simulink model "ANN"  (R2021b)
settings: Solver=FixedStepDiscrete  StartTime=0.0  StopTime=1  RelTol=1e-3
undefined symbols (not defined in the file or in its folder): alpha, b1, b2, b3, input, target, train, w1, w2, w3
Description:
  | Symmetric FIR Filter
  | This example shows how to use HDL Coder(TM) to check, generate,
  | and verify HDL for a fixed-point symmetric FIR filter.
settings Model: DataTypeOverride=Off  Creator=The MathWorks, Inc.  LastModifiedBy=bogru
settings SolverCC: AlgebraicLoopSolver=TrustRegion
settings DataIOCC: LimitDataPoints=on  SaveFormat=Array  SaveOutput=off  SignalLogging=off  SaveTime=off  ReturnWorkspaceOutputs=off  SignalLoggingName=logsOut
settings OptimizationCC: BlockReduction=off  BooleanDataType=off  ConditionallyExecuteInputs=off  DefaultParameterBehavior=Inlined  InheritOutputTypeSmallerThanSingle=on  InlineInvariantSignals=on  ExpressionDepthLimit=2147483647  InitFltsAndDblsToZero=on  LifeSpan=inf  BufferReusableBoundary=off
settings DebuggingCC: AlgebraicLoopMsg=error  SaveWithParameterizedLinksMsg=none  UnderspecifiedInitializationDetection=Classic  MergeDetectMultiDrivingBlocksExec=none  CheckExecutionContextPreStartOutputMsg=on  SignalResolutionControl=TryResolveAllWithWarning  MultiTaskDSMMsg=warning  MultiTaskCondExecSysMsg=none  SingleTaskRateTransMsg=error  IntegerOverflowMsg=none  ParameterPrecisionLossMsg=none  FcnCallInpInsideContextMsg=warning  BusObjectLabelMismatch=none  StateNameClashWarn=warning  SFUnexpectedBacktrackingDiag=warning  SFNoUnconditionalDefaultTransitionDiag=warning  SFExecutionAtInitializationDiag=none  SFMachineParentedDataDiag=warning  IntegerSaturationMsg=none  ArithmeticOperatorsInVariantConditions=warning
settings HardwareCC: ProdBitPerPointer=32  ProdBitPerSizeT=32  ProdBitPerPtrDiffT=32  ProdLargestAtomicFloat=None  ProdIntDivRoundTo=Undefined  ProdEndianess=Unspecified  ProdWordSize=32  ProdHWDeviceType=ASIC/FPGA  TargetUnknown=on  ProdEqTarget=off
settings ModelReferenceCC: PropagateSignalLabelsOutOfModel=off
settings SFSimCC: SimUseLocalCustomCode=off  CustomCodeUndefinedFunction=UseInterfaceOnly
settings RTWCC: RTWUseLocalCustomCode=off
settings CodeAppCC: StateflowObjectComments=on
settings GRTTargetCC: TargetFcnLib=ansi_tfl_tmw.mat  TargetLangStandard=C89/C90 (ANSI)  CombineOutputUpdateFcns=off  GRTInterface=on
settings ConfigComp: CovMetricSettings=dw  CovSaveCumulativeToWorkspaceVar=on  CovSaveSingleToWorkspaceVar=on  CovExternalEMLEnable=off

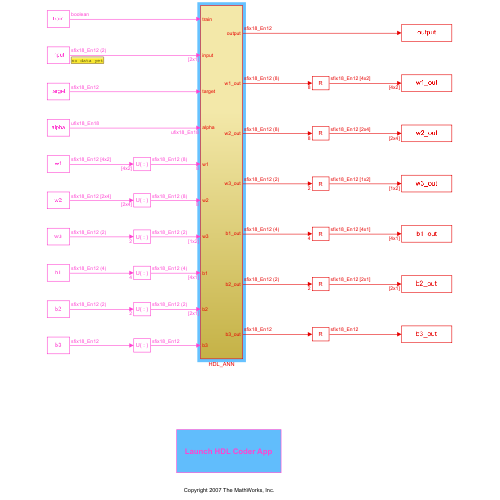
[thumbnail: Simulink's stored preview of the top-level diagram]
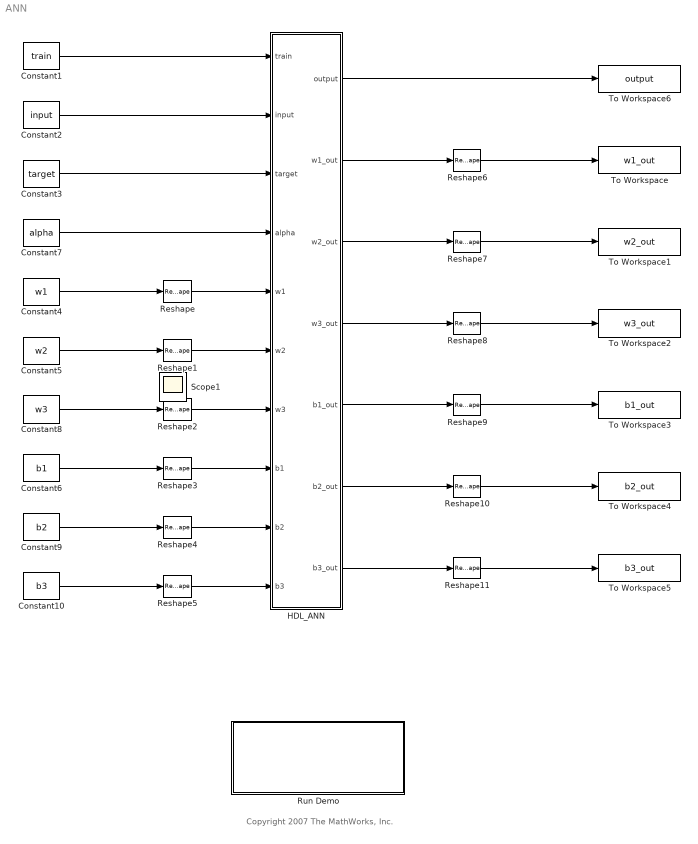
== system ANN ==
  note: Copyright 2007 The MathWorks, Inc.
  Constant1 : Constant  Value=train  OutDataTypeStr=boolean
  Constant10 : Constant  Value=b3  OutDataTypeStr=fixdt(1,18,12)
  Constant2 : Constant  Value=input  OutDataTypeStr=fixdt(1,18,12)
  Constant3 : Constant  Value=target  OutDataTypeStr=fixdt(1,18,12)
  Constant4 : Constant  Value=w1  OutDataTypeStr=fixdt(1,18,12)
  Constant5 : Constant  Value=w2  OutDataTypeStr=fixdt(1,18,12)
  Constant6 : Constant  Value=b1  OutDataTypeStr=fixdt(1,18,12)
  Constant7 : Constant  Value=alpha  OutDataTypeStr=fixdt(0,18,18)
  Constant8 : Constant  Value=w3  OutDataTypeStr=fixdt(1,18,12)
  Constant9 : Constant  Value=b2  OutDataTypeStr=fixdt(1,18,12)
  HDL_ANN : Subsystem
  Reshape{,1..5} (6 alike) : Reshape
  Reshape10 : Reshape  OutputDimensionality=Customize  OutputDimensions=[2 1]
  Reshape11 : Reshape  OutputDimensionality=Customize  OutputDimensions=[1 1]
  Reshape6 : Reshape  OutputDimensionality=Customize  OutputDimensions=[4 2]
  Reshape7 : Reshape  OutputDimensionality=Customize  OutputDimensions=[2 4]
  Reshape8 : Reshape  OutputDimensionality=Customize  OutputDimensions=[1 2]
  Reshape9 : Reshape  OutputDimensionality=Customize  OutputDimensions=[4 1]
  Run Demo : Subsystem
      settings: OpenFcn=hdltoolstrip(bdroot)
      mask Display: disp('Launch HDL Coder App')
  To Workspace : ToWorkspace  VariableName=w1_out  SampleTime=-1
      settings: MaxDataPoints=1
  To Workspace1 : ToWorkspace  VariableName=w2_out  SampleTime=-1
      settings: MaxDataPoints=1
  To Workspace2 : ToWorkspace  VariableName=w3_out  SampleTime=-1
      settings: MaxDataPoints=1
  To Workspace3 : ToWorkspace  VariableName=b1_out  SampleTime=-1
      settings: MaxDataPoints=1
  To Workspace4 : ToWorkspace  VariableName=b2_out  SampleTime=-1
      settings: MaxDataPoints=1
  To Workspace5 : ToWorkspace  VariableName=b3_out  SampleTime=-1
      settings: MaxDataPoints=1  Save2DSignal=2-D array (concatenate along first dimension)
  To Workspace6 : ToWorkspace  VariableName=output  SampleTime=-1
      settings: MaxDataPoints=1  Save2DSignal=2-D array (concatenate along first dimension)
  Scope1 : Scope
  wires:
  HDL_ANN/1(output) -> To Workspace6/1
  Constant7/1 -> HDL_ANN/4(alpha)
  Constant1/1 -> HDL_ANN/1(train)
  Constant3/1 -> HDL_ANN/3(target)
  Constant2/1 -> HDL_ANN/2(input)
  Constant4/1 -> Reshape/1
  Constant10/1 -> Reshape5/1
  Constant9/1 -> Reshape4/1
  Constant6/1 -> Reshape3/1
  Constant8/1 -> Reshape2/1
  Constant5/1 -> Reshape1/1
  HDL_ANN/2(w1_out) -> Reshape6/1
  Reshape/1 -> HDL_ANN/5(w1)
  Reshape1/1 -> HDL_ANN/6(w2)
  Reshape2/1 -> HDL_ANN/7(w3)
  Reshape3/1 -> HDL_ANN/8(b1)
  Reshape4/1 -> HDL_ANN/9(b2)
  Reshape5/1 -> HDL_ANN/10(b3)
  Reshape6/1 -> To Workspace/1
  HDL_ANN/3(w2_out) -> Reshape7/1
  Reshape7/1 -> To Workspace1/1
  HDL_ANN/4(w3_out) -> Reshape8/1
  Reshape8/1 -> To Workspace2/1
  HDL_ANN/5(b1_out) -> Reshape9/1
  Reshape9/1 -> To Workspace3/1
  HDL_ANN/6(b2_out) -> Reshape10/1
  Reshape10/1 -> To Workspace4/1
  HDL_ANN/7(b3_out) -> Reshape11/1
  Reshape11/1 -> To Workspace5/1

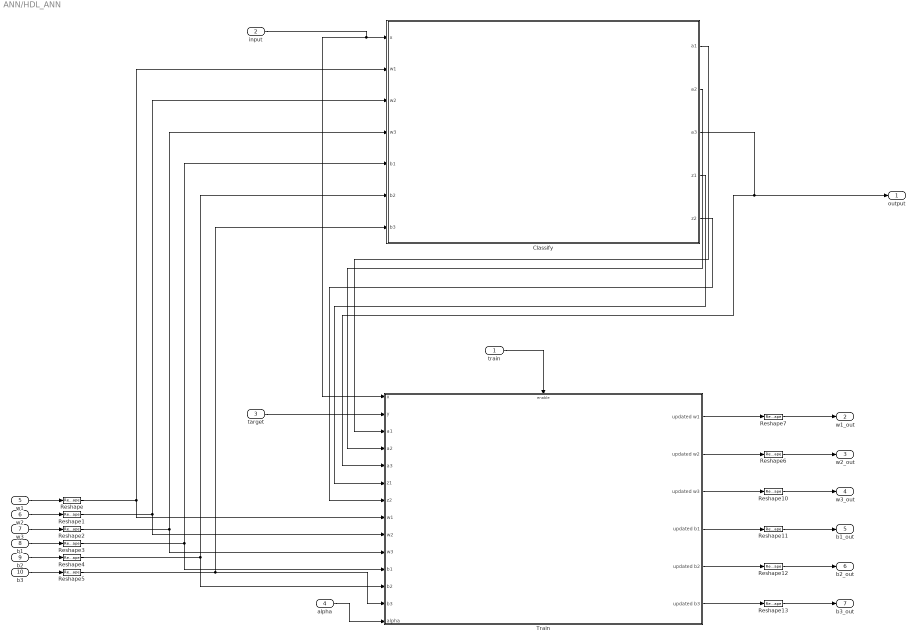
== system ANN/HDL_ANN ==
  train : Inport  SampleTime=1
  input : Inport  Port=2  PortDimensions=[2 1]  SampleTime=1
  target : Inport  Port=3  SampleTime=1
  alpha : Inport  Port=4  OutDataTypeStr=fixdt(0, 18, 18)  SampleTime=1
  w1 : Inport  Port=5  SampleTime=1
  w2 : Inport  Port=6  SampleTime=1
  w3 : Inport  Port=7  PortDimensions=[1 2]  SampleTime=1
  b1 : Inport  Port=8  PortDimensions=[4 1]  SampleTime=1
  b2 : Inport  Port=9  PortDimensions=[2 1]  SampleTime=1
  b3 : Inport  Port=10  PortDimensions=[1 1]  SampleTime=1
  Classify : Subsystem  TreatAsAtomicUnit=on
  Reshape : Reshape  OutputDimensionality=Customize  OutputDimensions=[4 2]
  Reshape1 : Reshape  OutputDimensionality=Customize  OutputDimensions=[2 4]
  Reshape{6..7,10..13} (6 alike) : Reshape  OutputDimensions=[4 2]
  Reshape2 : Reshape  OutputDimensionality=Customize  OutputDimensions=[1 2]
  Reshape3 : Reshape  OutputDimensionality=Customize  OutputDimensions=[4 1]
  Reshape4 : Reshape  OutputDimensionality=Customize  OutputDimensions=[2 1]
  Reshape5 : Reshape  OutputDimensionality=Customize  OutputDimensions=[1 1]
  Train : Subsystem  TreatAsAtomicUnit=on
  output : Outport
  w1_out : Outport  Port=2
  w2_out : Outport  Port=3
  w3_out : Outport  Port=4
  b1_out : Outport  Port=5
  b2_out : Outport  Port=6
  b3_out : Outport  Port=7
  wires:
  alpha/1 -> Train/14(alpha)
  Classify/2(a2) -> Train/4(a2)
  Classify/1(a1) -> Train/3(a1)
  Classify/3(a3) -> output/1, Train/5(a3)
  input/1 -> Train/1(x), Classify/1(x)
  target/1 -> Train/2(y)
  train/1 -> Train/Enable
  b3/1 -> Reshape5/1
  b2/1 -> Reshape4/1
  b1/1 -> Reshape3/1
  w3/1 -> Reshape2/1
  w1/1 -> Reshape/1
  Train/6(updated b3) -> Reshape13/1
  Train/5(updated b2) -> Reshape12/1
  Train/4(updated b1) -> Reshape11/1
  Train/3(updated w3) -> Reshape10/1
  Train/2(updated w2) -> Reshape6/1
  Train/1(updated w1) -> Reshape7/1
  Reshape/1 -> Classify/2(w1), Train/8(w1)
  Reshape1/1 -> Classify/3(w2), Train/9(w2)
  Reshape2/1 -> Classify/4(w3), Train/10(w3)
  Reshape3/1 -> Classify/5(b1), Train/11(b1)
  Reshape4/1 -> Classify/6(b2), Train/12(b2)
  Reshape5/1 -> Classify/7(b3), Train/13(b3)
  Reshape7/1 -> w1_out/1
  Reshape6/1 -> w2_out/1
  Reshape10/1 -> w3_out/1
  Reshape11/1 -> b1_out/1
  Reshape12/1 -> b2_out/1
  Reshape13/1 -> b3_out/1
  w2/1 -> Reshape1/1
  Classify/4(z1) -> Train/6(z1)
  Classify/5(z2) -> Train/7(z2)

== system ANN/Run Demo ==

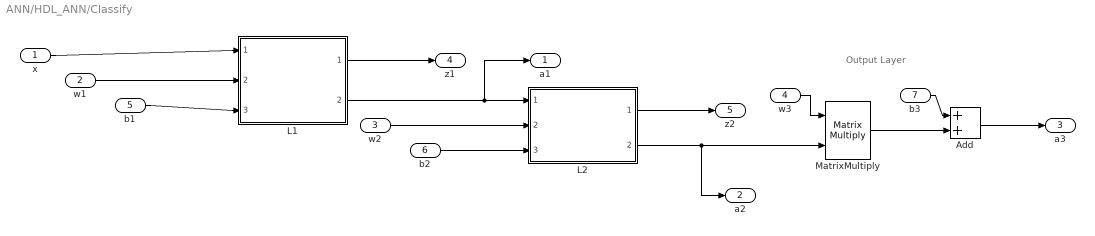
== system ANN/HDL_ANN/Classify ==
  note: Output Layer
  x : Inport
  w1 : Inport  Port=2
  w2 : Inport  Port=3
  w3 : Inport  Port=4
  b1 : Inport  Port=5
  b2 : Inport  Port=6
  b3 : Inport  Port=7
  Add : Sum  AccumDataTypeStr=fixdt(1,18,12)
  L1 : Subsystem  VariantControl=Choice  ReferencedSubsystem=ReLU_layer
  L2 : Subsystem  ReferencedSubsystem=ReLU_layer
  MatrixMultiply : Product  Multiplication=Matrix(*)  OutDataTypeStr=fixdt(1,18,12)
  a1 : Outport  InitialOutput=[0;0;0;0]
  a2 : Outport  Port=2  InitialOutput=[0;0]
  a3 : Outport  Port=3  InitialOutput=0
  z1 : Outport  Port=4  InitialOutput=[0;0;0;0]
  z2 : Outport  Port=5  InitialOutput=[0;0;0;0]
  wires:
  w2/1 -> L2/2
  b2/1 -> L2/3
  x/1 -> L1/1
  w1/1 -> L1/2
  b1/1 -> L1/3
  L1/1 -> z1/1
  L1/2 -> a1/1, L2/1
  L2/1 -> z2/1
  w3/1 -> MatrixMultiply/1
  L2/2 -> MatrixMultiply/2, a2/1
  b3/1 -> Add/1
  MatrixMultiply/1 -> Add/2
  Add/1 -> a3/1

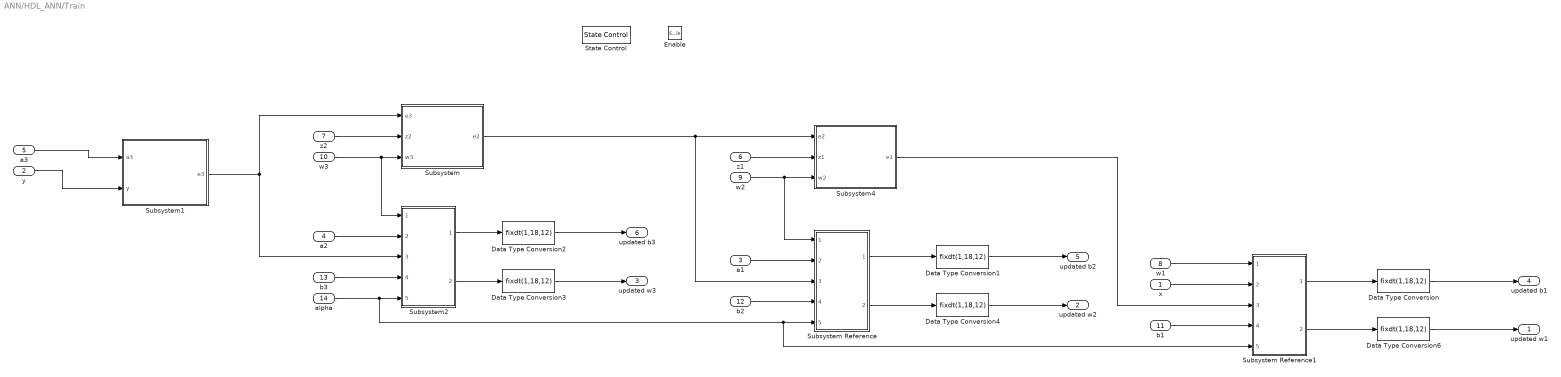
== system ANN/HDL_ANN/Train ==
  x : Inport
  y : Inport  Port=2
  a1 : Inport  Port=3
  a2 : Inport  Port=4
  a3 : Inport  Port=5
  z1 : Inport  Port=6
  z2 : Inport  Port=7
  w1 : Inport  Port=8
  w2 : Inport  Port=9
  w3 : Inport  Port=10
  b1 : Inport  Port=11
  b2 : Inport  Port=12
  b3 : Inport  Port=13
  alpha : Inport  Port=14
  Enable : EnablePort
  Data Type Conversion{,1..4,6} (6 alike) : DataTypeConversion  OutDataTypeStr=fixdt(1,18,12)
  State Control : StateControl  StateControl=Synchronous
  Subsystem : Subsystem
  Subsystem Reference : Subsystem  ReferencedSubsystem=WB_update
  Subsystem Reference1 : Subsystem  ReferencedSubsystem=WB_update
  Subsystem1 : Subsystem
  Subsystem2 : Subsystem  ReferencedSubsystem=WB_update
  Subsystem4 : Subsystem
  updated w1 : Outport  InitialOutput=[0 0; 0 0; 0 0; 0 0]
  updated w2 : Outport  Port=2  InitialOutput=[0 0 0 0; 0 0 0 0]
  updated w3 : Outport  Port=3  InitialOutput=[0 0]
  updated b1 : Outport  Port=4  InitialOutput=[0;0;0;0]
  updated b2 : Outport  Port=5  InitialOutput=[0;0]
  updated b3 : Outport  Port=6  InitialOutput=0
  wires:
  Data Type Conversion6/1 -> updated w1/1
  Subsystem4/1(e1) -> Subsystem Reference1/3
  Subsystem Reference1/2 -> Data Type Conversion6/1
  Data Type Conversion4/1 -> updated w2/1
  Subsystem/1(e2) -> Subsystem Reference/3, Subsystem4/1(e2)
  Data Type Conversion3/1 -> updated w3/1
  Subsystem2/2 -> Data Type Conversion3/1
  Data Type Conversion1/1 -> updated b2/1
  Data Type Conversion2/1 -> updated b3/1
  w2/1 -> Subsystem Reference/1, Subsystem4/3(w2)
  a1/1 -> Subsystem Reference/2
  b1/1 -> Subsystem Reference1/4
  b3/1 -> Subsystem2/4
  w1/1 -> Subsystem Reference1/1
  b2/1 -> Subsystem Reference/4
  Data Type Conversion/1 -> updated b1/1
  Subsystem Reference1/1 -> Data Type Conversion/1
  a2/1 -> Subsystem2/2
  x/1 -> Subsystem Reference1/2
  w3/1 -> Subsystem2/1, Subsystem/3(w3)
  Subsystem Reference/1 -> Data Type Conversion1/1
  Subsystem2/1 -> Data Type Conversion2/1
  alpha/1 -> Subsystem2/5, Subsystem Reference1/5, Subsystem Reference/5
  Subsystem Reference/2 -> Data Type Conversion4/1
  z1/1 -> Subsystem4/2(z1)
  z2/1 -> Subsystem/2(z2)
  Subsystem1/1(e3) -> Subsystem/1(e3), Subsystem2/3
  a3/1 -> Subsystem1/1(a3)
  y/1 -> Subsystem1/2(y)

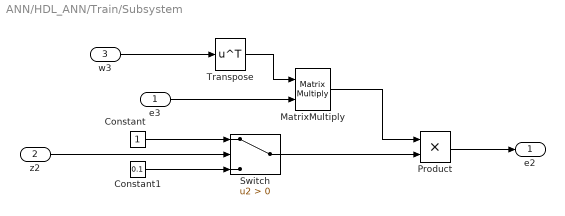
== system ANN/HDL_ANN/Train/Subsystem ==
  e3 : Inport
  z2 : Inport  Port=2
  w3 : Inport  Port=3
  Constant : Constant  OutDataTypeStr=fixdt(1,18,12)  SampleTime=-1
  Constant1 : Constant  Value=0.1  OutDataTypeStr=fixdt(1,18,12)  SampleTime=-1
  MatrixMultiply : Product  Multiplication=Matrix(*)
  Product : Product
  Switch : Switch  Criteria=u2 > Threshold
  Transpose : Math  Operator=transpose  SaturateOnIntegerOverflow=on
  e2 : Outport
  wires:
  w3/1 -> Transpose/1
  Transpose/1 -> MatrixMultiply/1
  e3/1 -> MatrixMultiply/2
  Product/1 -> e2/1
  Constant/1 -> Switch/1
  Constant1/1 -> Switch/3
  z2/1 -> Switch/2
  MatrixMultiply/1 -> Product/1
  Switch/1 -> Product/2

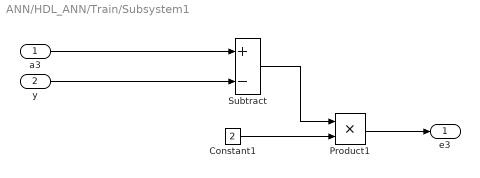
== system ANN/HDL_ANN/Train/Subsystem1 ==
  a3 : Inport
  y : Inport  Port=2
  Constant1 : Constant  Value=2  OutDataTypeStr=fixdt(1,18,12)  SampleTime=-1
  Product1 : Product
  Subtract : Sum  Inputs=+-
  e3 : Outport
  wires:
  y/1 -> Subtract/2
  a3/1 -> Subtract/1
  Product1/1 -> e3/1
  Subtract/1 -> Product1/1
  Constant1/1 -> Product1/2

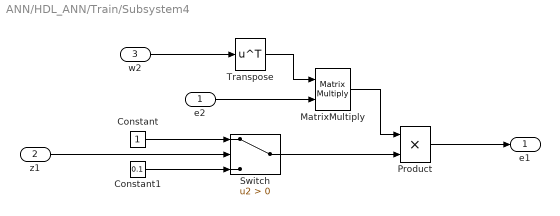
== system ANN/HDL_ANN/Train/Subsystem4 ==
  e2 : Inport
  z1 : Inport  Port=2
  w2 : Inport  Port=3
  Constant : Constant  OutDataTypeStr=fixdt(1,18,12)  SampleTime=-1
  Constant1 : Constant  Value=0.1  OutDataTypeStr=fixdt(1,18,12)  SampleTime=-1
  MatrixMultiply : Product  Multiplication=Matrix(*)
  Product : Product  OutDataTypeStr=Inherit: Inherit via back propagation
  Switch : Switch  Criteria=u2 > Threshold
  Transpose : Math  Operator=transpose  SaturateOnIntegerOverflow=on
  e1 : Outport
  wires:
  w2/1 -> Transpose/1
  Transpose/1 -> MatrixMultiply/1
  e2/1 -> MatrixMultiply/2
  MatrixMultiply/1 -> Product/1
  Product/1 -> e1/1
  z1/1 -> Switch/2
  Switch/1 -> Product/2
  Constant/1 -> Switch/1
  Constant1/1 -> Switch/3
